simulink model "sidemission_model"  (R2018b)
settings: Solver=ode3  StartTime=0.0  StopTime=10  RelTol=1e-3  EnableMultiTasking=on
libraries: legoev3lib x10
settings Model: FPTRunName=Active  ExtModeTrigDuration=2  Creator=jloehnertz  LastModifiedBy=jloehnertz
settings SolverCC: PositivePriorityOrder=on
settings DataIOCC: LimitDataPoints=on  SaveFormat=Array
settings OptimizationCC: ExpressionDepthLimit=2147483647  LifeSpan=Inf  MaxStackSize=64
settings DebuggingCC: UnderspecifiedInitializationDetection=Classic  MergeDetectMultiDrivingBlocksExec=none  FcnCallInpInsideContextMsg=warning  AllowSymbolicDim=off  StateNameClashWarn=warning  SFUnexpectedBacktrackingDiag=warning  SFNoUnconditionalDefaultTransitionDiag=warning  SFExecutionAtInitializationDiag=none
settings HardwareCC: ProdBitPerPointer=32  ProdBitPerSizeT=32  ProdBitPerPtrDiffT=32  ProdLargestAtomicInteger=Long  ProdWordSize=32  ProdHWDeviceType=ARM Compatible->ARM 9  UseEmbeddedCoderFeatures=off  UseSimulinkCoderFeatures=off
settings ModelReferenceCC: PropagateSignalLabelsOutOfModel=off
settings SFSimCC: SimUseLocalCustomCode=off
settings RTWCC: SystemTargetFile=ert.tlc  HardwareBoard=LEGO MINDSTORMS EV3  TemplateMakefile=ert_default_tmf  GenerateReport=on  RTWVerbose=off  RTWUseLocalCustomCode=off  Toolchain=Sourcery G++ Lite v2009q3  BuildConfiguration=Faster Runs  LaunchReport=on
settings CodeAppCC: ForceParamTrailComments=on  OperatorAnnotations=on  StateflowObjectComments=on  MATLABSourceComments=on
settings ERTTargetCC: MultiwordLength=2048  ERTCustomFileBanners=off  SupportContinuousTime=on  SupportNonInlinedSFcns=on  RemoveResetFunc=off  SupportVariableSizeSignals=on  ModelStepFunctionPrototypeControlCompliant=off
settings ConfigComp: CovMetricSettings=dw  CovHtmlReporting=on  CovSaveCumulativeToWorkspaceVar=on  CovSaveSingleToWorkspaceVar=on  CovExternalEMLEnable=off  CovSFcnEnable=off

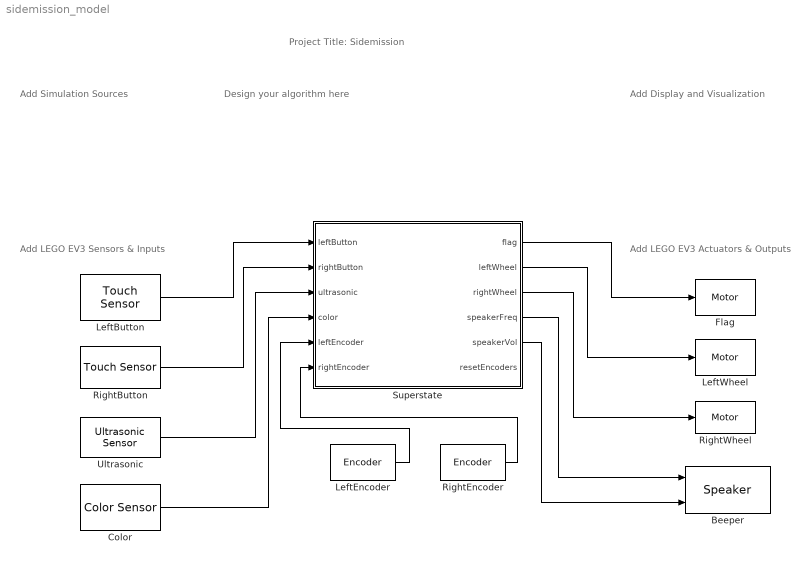
== system sidemission_model ==
  note: Add LEGO EV3 Sensors & Inputs
  note: Add Display and Visualization
  note: Design your algorithm here
  note: Add LEGO EV3 Actuators & Outputs
  note: Add Simulation Sources
  note: Project Title: Sidemission
  Beeper : legoev3lib/Speaker  sinputMode=Frequency and volume  sspeakerFreq=100  sspeakerVolume=50  sspeakerDuration=100
      settings: SourceProductName=Simulink Support Package for LEGO MINDSTORMS EV3 Hardware  SourceProductBaseCode=LEGOEV3
  Color : legoev3lib/Color Sensor  portNumber=3  mode=Color  sampleTime=0.1
      settings: SourceProductName=Simulink Support Package for LEGO MINDSTORMS EV3 Hardware  SourceProductBaseCode=LEGOEV3
  Flag : legoev3lib/Motor  sportNumber=A  sstopAction=Brake
  LeftButton : legoev3lib/Touch Sensor  portNumber=1  sampleTime=0.1
      settings: SourceProductName=Simulink Support Package for LEGO MINDSTORMS EV3 Hardware  SourceProductBaseCode=LEGOEV3
  LeftEncoder : legoev3lib/Encoder  portNumber=C  opMode=Reset by external signal  sampleTime=0.1
      settings: SourceProductName=Simulink Support Package for LEGO MINDSTORMS EV3 Hardware  SourceProductBaseCode=LEGOEV3
  LeftWheel : legoev3lib/Motor  sportNumber=C  sstopAction=Brake
  RightButton : legoev3lib/Touch Sensor  portNumber=2  sampleTime=0.1
      settings: SourceProductName=Simulink Support Package for LEGO MINDSTORMS EV3 Hardware  SourceProductBaseCode=LEGOEV3
  RightEncoder : legoev3lib/Encoder  portNumber=B  opMode=Reset by external signal  sampleTime=0.1
      settings: SourceProductName=Simulink Support Package for LEGO MINDSTORMS EV3 Hardware  SourceProductBaseCode=LEGOEV3
  RightWheel : legoev3lib/Motor  sportNumber=B  sstopAction=Brake
  Superstate : Stateflow chart  TreatAsAtomicUnit=on
  Ultrasonic : legoev3lib/Ultrasonic Sensor  PortNumber=4  sampleTime=0.1
      settings: SourceProductName=Simulink Support Package for LEGO MINDSTORMS EV3 Hardware  SourceProductBaseCode=LEGOEV3
  wires:
  Superstate/5(speakerVol) -> Beeper/2
  RightEncoder/1 -> Superstate/6(rightEncoder)
  Superstate/2(leftWheel) -> LeftWheel/1
  Superstate/3(rightWheel) -> RightWheel/1
  LeftEncoder/1 -> Superstate/5(leftEncoder)
  Superstate/4(speakerFreq) -> Beeper/1
  Superstate/1(flag) -> Flag/1
  Color/1 -> Superstate/4(color)
  Ultrasonic/1 -> Superstate/3(ultrasonic)
  LeftButton/1 -> Superstate/1(leftButton)
  RightButton/1 -> Superstate/2(rightButton)

== stateflow chart sidemission_model/Superstate ==
  state Sidemission
    state Do360NoScope
      entry:
      startRotation = rightEncoder - leftEncoder;
      speakerFreq = 0;
      speakerVol = 0;
      leftWheel = -scanSpeed;
      rightWheel = scanSpeed;
      state UpdateNearestObstacle
        entry:
        rotationNearestObstacle = rightEncoder - leftEncoder;
      state FindNearestObstacle
      state ResetEncoders
        entry:
        resetEncoders = 1;
        exit:
        resetEncoders = 0;
      state Stop
        entry:
        leftWheel = 0;
        rightWheel = 0;
      FindNearestObstacle -> UpdateNearestObstacle [order 1] : [ultrasonic < distanceNearestObstacle]
      (default) -> ResetEncoders
      ResetEncoders -> FindNearestObstacle : after(0.1, sec)
      UpdateNearestObstacle -> FindNearestObstacle
      FindNearestObstacle -> Stop [order 2] : [leftEncoder - rightEncoder >= 3.8 * 360 - startRotation]
    (default) -> Do360NoScope
  state Manual
    state RESET
    state AUTONOMOUS
      entry:
      send(startAutonomous)
    state TURNLEFT
      entry:
      leftWheel = 23
      rightWheel = -23
    state MANUAL
      entry:
      leftWheel = 0;
      rightWheel = 0;
    state HOLD
    state WAIT
    state STOP
    state FORWARD
      entry:
      leftWheel = 30;
      rightWheel = 30;
    state SIDEMISSION
      entry:
      send(startSidemission)
    state TURNRIGHT
      entry:
      leftWheel = -23
      rightWheel = 23
    RESET -> MANUAL [order 1] : after(1, sec)
    RESET -> AUTONOMOUS [order 2] : [not(leftButton == 1 & rightButton == 1)]
    TURNLEFT -> MANUAL : [not(leftButton == 1 & rightButton == 0)]
    MANUAL -> TURNLEFT [order 1] : [leftButton == 1 & rightButton == 0]
    WAIT -> AUTONOMOUS [order 2] : [not(leftButton == 1 & rightButton == 1)]
    (default) -> MANUAL
    HOLD -> WAIT [order 2] : after(1, sec)
    MANUAL -> HOLD [order 3] : [leftButton == 1 & rightButton == 1]
    HOLD -> FORWARD [order 1] : [not(leftButton == 1 & rightButton == 1)]
    WAIT -> SIDEMISSION [order 1] : after(2, sec)
    STOP -> MANUAL : [leftButton == 0 & rightButton == 0]
    FORWARD -> STOP : [not(leftButton == 0 & rightButton == 0)]
    TURNRIGHT -> MANUAL : [not(leftButton == 0 & rightButton == 1)]
    MANUAL -> TURNRIGHT [order 2] : [leftButton == 0 & rightButton == 1]
  (default) -> Manual
  Manual -> Sidemission : [startSidemission]
  data: leftButton input; rightButton input; flag output =0; leftWheel output; rightWheel output; speakerFreq output; speakerVol output; ultrasonic input; color input; stopDistance constant double =15; resetEncoders output; leftEncoder input; rightEncoder input; driveSpeed constant double =50; lastDirection local =0; scanSpeed constant double =25; waitTime local; desiredSpeakerVol constant double =55; turnDirectionAfterFleeing local =0; rotationNearestObstacle local; startRotation local; distanceNearestObstacle local =100
  events: startFlee local FUNCTION_CALL_EVENT; startAutonomous local FUNCTION_CALL_EVENT; initLineFollow local FUNCTION_CALL_EVENT; startLineFollow local FUNCTION_CALL_EVENT; startSidemission local FUNCTION_CALL_EVENT
